simulink model "CounterCondition"  (R2020b)
settings: Solver=VariableStepAuto  StartTime=0.0  StopTime=10.0  RelTol=1e-3
settings Model: Creator=90546  LastModifiedBy=90546

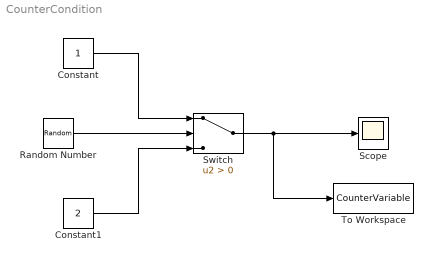
== system CounterCondition ==
  Constant : Constant
  Constant1 : Constant  Value=2
  Random Number : RandomNumber  SampleTime=0.1
  Scope : Scope
  Switch : Switch  Criteria=u2 > Threshold
  To Workspace : ToWorkspace  VariableName=CounterVariable  SaveFormat=Timeseries  SampleTime=-1
  wires:
  Random Number/1 -> Switch/2
  Switch/1 -> To Workspace/1, Scope/1
  Constant/1 -> Switch/1
  Constant1/1 -> Switch/3
